simulink model "FDIlinkSimulinkSerial_20231225"  (R2022a)
settings: Solver=VariableStepAuto  StartTime=0.0  StopTime=inf  RelTol=1e-3
libraries: instrumentseriallib x2, aerolibconvert2 x1, sharedtransform x1
settings Model: Creator=JackyL  LastModifiedBy=Administrator
settings SolverCC: AlgebraicLoopSolver=TrustRegion
settings DataIOCC: ReturnWorkspaceOutputs=off
settings DebuggingCC: UnconnectedInputMsg=warning  UnconnectedOutputMsg=warning  UnconnectedLineMsg=warning  SFMachineParentedDataDiag=warning  ArithmeticOperatorsInVariantConditions=warning
settings SFSimCC: CustomCodeUndefinedFunction=UseInterfaceOnly
settings RTWCC: DLArmComputeVersion=19.05

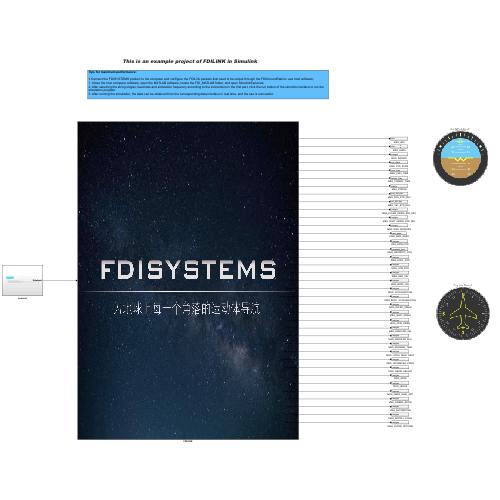
[thumbnail: Simulink's stored preview of the top-level diagram]
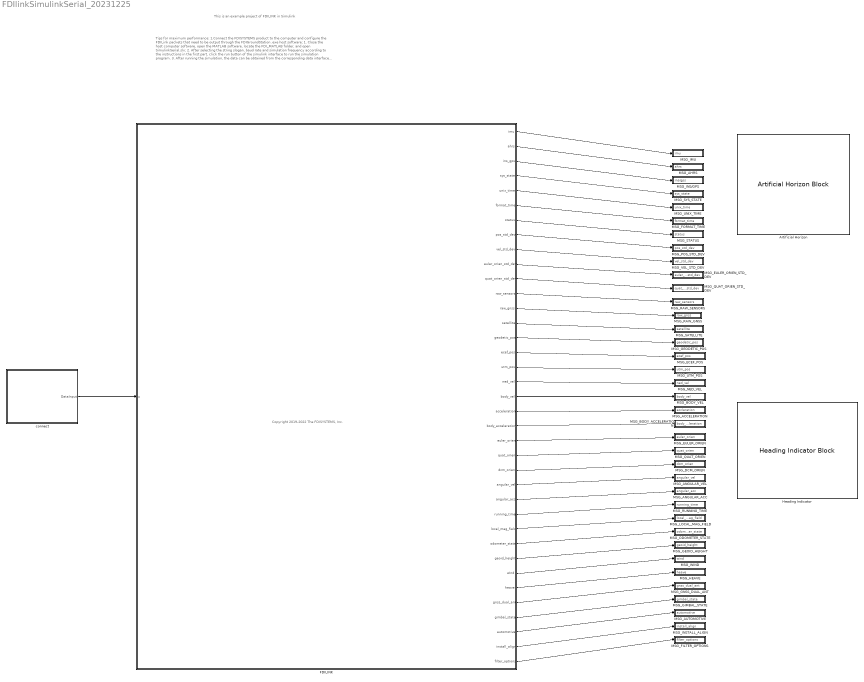
== system FDIlinkSimulinkSerial_20231225 ==
  note: This is an example project of FDILINK in Simulink
  note: Copyright 2019-2022 The FDISYSTEMS, Inc.
  note: Tips for maximum performance:
      |
      | 1.Connect the FDISYSTEMS product to the computer and configure the FDILink packets that need to be output through the FDIGroundStation .exe host software;
      | 1. Close the host computer software, open the MATLAB software, locate the FDI_MATLAB folder, and open SimulinkSerial.slx;
      | 2. After selecting the string slogan, baud rate and simulation frequency according to the instructions in the first part, click the run button of the simulink interface to run the simulation program.
      | 3. After running the simulation, the data can be obtained from the corresponding data interface in real time, and the use is successful.
      |
      | Secondary development: You can follow the example program in the following FDILINK module, add the data that needs to be parsed, specifically need to refer to the fdilink protocol document to write, and finally, pay attention to the computer software to enable this data frame.
  Artificial Horizon : ArtificialHorizonBlock
  FDILINK : MATLAB Function  TreatAsAtomicUnit=on
  Heading Indicator : HeadingIndicatorBlock
  MSG_ACCELERATION : Subsystem
  "MSG_AHRS " : Subsystem
  MSG_ANGULAR_ACC : Subsystem
  MSG_ANGULAR_VEL : Subsystem
  MSG_AUTOMOTIVE : Subsystem
  MSG_BODY_ACCELERATION : Subsystem
  MSG_BODY_VEL : Subsystem
  MSG_DCM_ORIEN : Subsystem
  MSG_ECEF_POS : Subsystem
  MSG_EULER_ORIEN : Subsystem
  MSG_EULER_ORIEN_STD_DEV : Subsystem
  MSG_FILTER_OPTIONS : Subsystem
  MSG_FORMAT_TIME : Subsystem
  MSG_GEODETIC_POS : Subsystem
  MSG_GEOID_HEIGHT : Subsystem
  MSG_GIMBAL_STATE : Subsystem
  MSG_GNSS_DUAL_ANT : Subsystem
  MSG_HEAVE : Subsystem
  "MSG_IMU " : Subsystem
  MSG_INS/GPS : Subsystem
  MSG_INSTALL_ALIGN : Subsystem
  MSG_LOCAL_MAG_FIELD : Subsystem
  MSG_NED_VEL : Subsystem
  MSG_ODOMETER_STATE : Subsystem
  MSG_POS_STD_DEV : Subsystem
  MSG_QUAT_ORIEN : Subsystem
  MSG_QUAT_ORIEN_STD_DEV : Subsystem
  MSG_RAW_GNSS : Subsystem
  MSG_RAW_SENSORS : Subsystem
  MSG_RUNNING_TIME : Subsystem
  MSG_SATELLITE : Subsystem
  MSG_STATUS : Subsystem
  MSG_SYS_STATE : Subsystem
  MSG_UNIX_TIME : Subsystem
  MSG_UTM_POS : Subsystem
  MSG_VEL_STD_DEV : Subsystem
  MSG_WIND : Subsystem
  connect : Subsystem
  wires:
  connect/1(DataInput) -> FDILINK/1(u)
  FDILINK/1(imu) -> "MSG_IMU "/1("imu ")
  FDILINK/2(ahrs) -> "MSG_AHRS "/1("ahrs ")
  FDILINK/3(ins_gps) -> MSG_INS/GPS/1("ins/gps ")
  FDILINK/13(raw_gnss) -> MSG_RAW_GNSS/1("raw_gnss ")
  FDILINK/15(geodetic_pos) -> MSG_GEODETIC_POS/1("geodetic_pos ")
  FDILINK/4(sys_state) -> MSG_SYS_STATE/1("sys_state ")
  FDILINK/5(unix_time) -> MSG_UNIX_TIME/1("unix_time ")
  FDILINK/6(format_time) -> MSG_FORMAT_TIME/1("format_time ")
  FDILINK/7(status) -> MSG_STATUS/1("status ")
  FDILINK/8(pos_std_dev) -> MSG_POS_STD_DEV/1("pos_std_dev ")
  FDILINK/9(vel_std_dev) -> MSG_VEL_STD_DEV/1("vel_std_dev ")
  FDILINK/10(euler_orien_std_dev) -> MSG_EULER_ORIEN_STD_DEV/1("euler_orien_std_dev ")
  FDILINK/11(quat_orien_std_dev) -> MSG_QUAT_ORIEN_STD_DEV/1("quat_orien_std_dev ")
  FDILINK/12(raw_sensors) -> MSG_RAW_SENSORS/1("raw_sensors ")
  FDILINK/14(satellite) -> MSG_SATELLITE/1("satellite ")
  FDILINK/16(ecef_pos) -> MSG_ECEF_POS/1("ecef_pos ")
  FDILINK/17(utm_pos) -> MSG_UTM_POS/1("utm_pos ")
  FDILINK/18(ned_vel) -> MSG_NED_VEL/1("ned_vel ")
  FDILINK/19(body_vel) -> MSG_BODY_VEL/1("body_vel ")
  FDILINK/20(acceleration) -> MSG_ACCELERATION/1("accleration ")
  FDILINK/21(body_acceleration) -> MSG_BODY_ACCELERATION/1("body_acceleration ")
  FDILINK/22(euler_orien) -> MSG_EULER_ORIEN/1("euler_orien ")
  FDILINK/23(quat_orien) -> MSG_QUAT_ORIEN/1("quat_orien ")
  FDILINK/24(dcm_orien) -> MSG_DCM_ORIEN/1("dcm_orien ")
  FDILINK/25(angular_vel) -> MSG_ANGULAR_VEL/1("angular_vel ")
  FDILINK/26(angular_acc) -> MSG_ANGULAR_ACC/1("angular_acc ")
  FDILINK/27(running_time) -> MSG_RUNNING_TIME/1("running_time ")
  FDILINK/28(local_mag_field) -> MSG_LOCAL_MAG_FIELD/1("local_mag_field ")
  FDILINK/29(odometer_state) -> MSG_ODOMETER_STATE/1("odometer_state ")
  FDILINK/30(geoid_height) -> MSG_GEOID_HEIGHT/1("geoid_height ")
  FDILINK/31(wind) -> MSG_WIND/1("wind ")
  FDILINK/32(heave) -> MSG_HEAVE/1("heave ")
  FDILINK/33(gnss_dual_ant) -> MSG_GNSS_DUAL_ANT/1("gnss_dual_ant ")
  FDILINK/34(gimbal_state) -> MSG_GIMBAL_STATE/1("gimbal_state ")
  FDILINK/35(automotive) -> MSG_AUTOMOTIVE/1("automotive ")
  FDILINK/36(install_align) -> MSG_INSTALL_ALIGN/1("install_align ")
  FDILINK/37(filter_options) -> MSG_FILTER_OPTIONS/1("filter_options ")

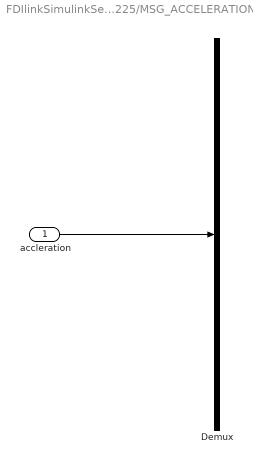
== system FDIlinkSimulinkSerial_20231225/MSG_ACCELERATION ==
  "accleration " : Inport
  Demux : Demux  Outputs=3
  wires:
  "accleration "/1 -> Demux/1

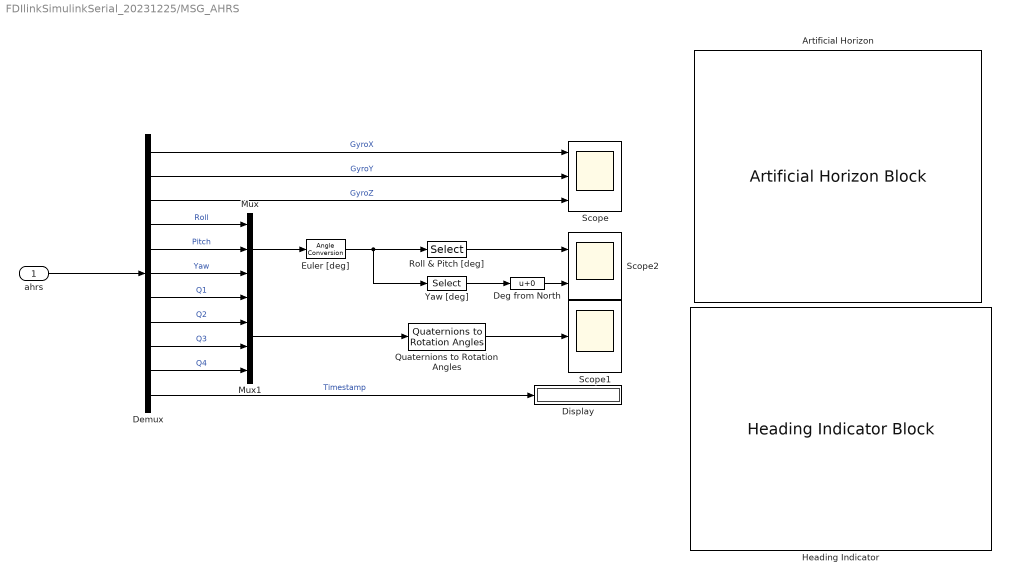
== system FDIlinkSimulinkSerial_20231225/MSG_AHRS  ==
  "ahrs " : Inport
  Artificial Horizon : ArtificialHorizonBlock
  Deg from North : Bias  SaturateOnIntegerOverflow=off
  Demux : Demux  Outputs=11
  Display : Display
  Euler [deg] : aerolibconvert2/Angle Conversion  IU=rad  OU=deg
  Heading Indicator : HeadingIndicatorBlock
  Mux : Mux  Inputs=3
  Mux1 : Mux
  Quaternions to Rotation Angles : sharedtransform/Quaternions to Rotation Angles  rotationOrder=ZYX  aMode=aMode
      settings: SourceProductBaseCode=AE,PW,DR,MT,VE
  Roll & Pitch [deg] : Selector  InputPortWidth=3  IndexOptions=Index vector (dialog)  Indices=[1 2]  OutputSizes=1
  Scope : Scope  NumInputPorts=3
  Scope1 : Scope
  Scope2 : Scope  NumInputPorts=2
  Yaw [deg] : Selector  InputPortWidth=3  IndexOptions=Index vector (dialog)  Indices=[3]  OutputSizes=1
  wires:
  "ahrs "/1 -> Demux/1
  Demux/1 -> Scope/1  "GyroX"
  Demux/2 -> Scope/2  "GyroY"
  Demux/3 -> Scope/3  "GyroZ"
  Demux/5 -> Mux/2  "Pitch"
  Demux/7 -> Mux1/1  "Q1"
  Demux/8 -> Mux1/2  "Q2"
  Demux/9 -> Mux1/3  "Q3"
  Demux/10 -> Mux1/4  "Q4"
  Demux/11 -> Display/1  "Timestamp"
  Demux/4 -> Mux/1  "Roll"
  Demux/6 -> Mux/3  "Yaw"
  Mux/1 -> Euler [deg]/1
  Euler [deg]/1 -> Yaw [deg]/1, Roll & Pitch [deg]/1
  Yaw [deg]/1 -> Deg from North/1
  Mux1/1 -> Quaternions to Rotation Angles/1
  Quaternions to Rotation Angles/1 -> Scope1/1
  Roll & Pitch [deg]/1 -> Scope2/1
  Deg from North/1 -> Scope2/2

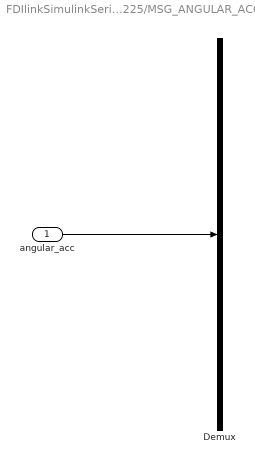
== system FDIlinkSimulinkSerial_20231225/MSG_ANGULAR_ACC ==
  "angular_acc " : Inport
  Demux : Demux  Outputs=3
  wires:
  "angular_acc "/1 -> Demux/1

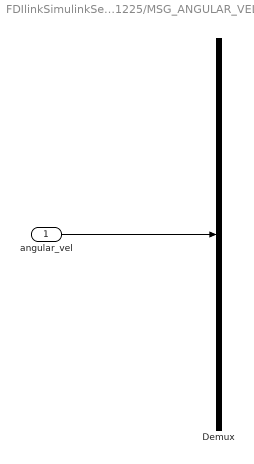
== system FDIlinkSimulinkSerial_20231225/MSG_ANGULAR_VEL ==
  "angular_vel " : Inport
  Demux : Demux  Outputs=3
  wires:
  "angular_vel "/1 -> Demux/1

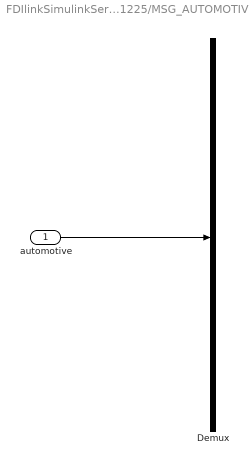
== system FDIlinkSimulinkSerial_20231225/MSG_AUTOMOTIVE ==
  "automotive " : Inport
  Demux : Demux  Outputs=6
  wires:
  "automotive "/1 -> Demux/1

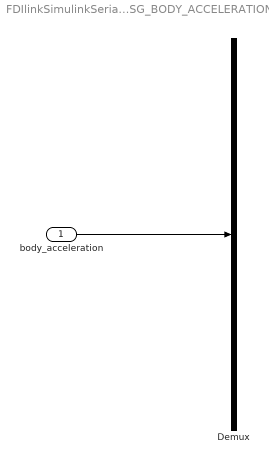
== system FDIlinkSimulinkSerial_20231225/MSG_BODY_ACCELERATION ==
  "body_acceleration " : Inport
  Demux : Demux
  wires:
  "body_acceleration "/1 -> Demux/1

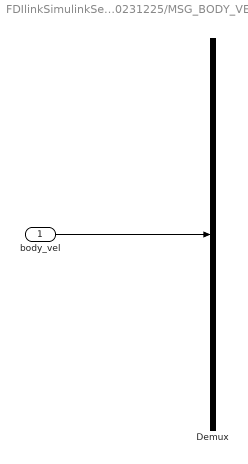
== system FDIlinkSimulinkSerial_20231225/MSG_BODY_VEL ==
  "body_vel " : Inport
  Demux : Demux  Outputs=3
  wires:
  "body_vel "/1 -> Demux/1

== system FDIlinkSimulinkSerial_20231225/MSG_DCM_ORIEN ==
  "dcm_orien " : Inport
  Demux : Demux  Outputs=9
  wires:
  "dcm_orien "/1 -> Demux/1

== system FDIlinkSimulinkSerial_20231225/MSG_ECEF_POS ==
  "ecef_pos " : Inport
  Demux : Demux  Outputs=3
  wires:
  "ecef_pos "/1 -> Demux/1

== system FDIlinkSimulinkSerial_20231225/MSG_EULER_ORIEN ==
  "euler_orien " : Inport
  Demux : Demux  Outputs=3
  wires:
  "euler_orien "/1 -> Demux/1

== system FDIlinkSimulinkSerial_20231225/MSG_EULER_ORIEN_STD_DEV ==
  "euler_orien_std_dev " : Inport
  Demux : Demux  Outputs=3
  wires:
  "euler_orien_std_dev "/1 -> Demux/1

== system FDIlinkSimulinkSerial_20231225/MSG_FILTER_OPTIONS ==
  "filter_options " : Inport
  Demux : Demux  Outputs=21
  wires:
  "filter_options "/1 -> Demux/1

== system FDIlinkSimulinkSerial_20231225/MSG_FORMAT_TIME ==
  "format_time " : Inport
  Demux : Demux  Outputs=9
  wires:
  "format_time "/1 -> Demux/1

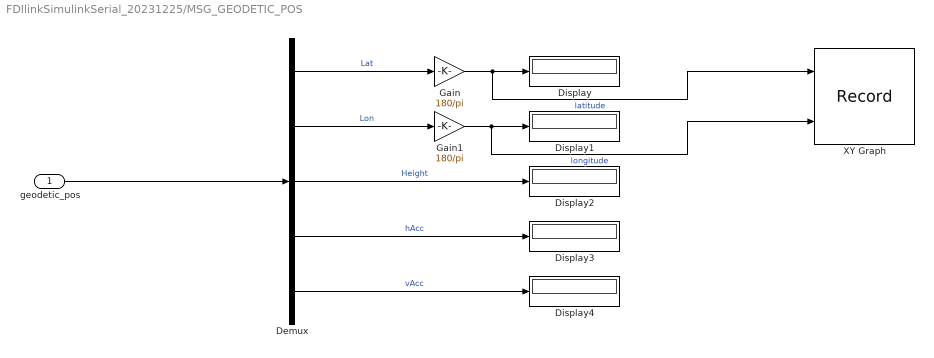
== system FDIlinkSimulinkSerial_20231225/MSG_GEODETIC_POS ==
  "geodetic_pos " : Inport
  Demux : Demux  Outputs=5
  Display{,1..4} (5 alike) : Display
  Gain : Gain  Gain=180/pi
  Gain1 : Gain  Gain=180/pi
  XY Graph : Record  FileSettingsInternal="{\"entries\":[{\"content\":{\"excelSettings\":{\"content\":{},\"type\":\"Streamout.ExcelSettings\"}},\"type\":\"Streamout.FileSettingStorage\",\"uuid\":\"c57b3c35-ac54-404b-860e-26f47809a26e\"}],\"packageUris\":[\"http://schema.mathworks.com/mf0/streamout_blocks/R2020a\"],\"version\":\"1.0\"}"  Layout=[1 1]  SignalsInternal="{\"entries\":[{\"content\":{\"signals\":[{\"content\":{\"blockPath\":[\"FDIlinkSimulinkSerial_2023/MSG_GEODETIC_POS/XY Graph\"],\"channel\":[],\"dimensions\":[1],\"domain\":\"FDIlinkSimulinkSerial_2023/MSG_GEODETIC_POS/XY Graph\",\"lineColor\":\"#a2142f\",\"plots\":[1],\"port\":1,\"sid\":[\"\"],\"signalID\":52640,\"signalName\":\"latitude\"},\"type\":\"RecordBlkView.Signal\",\"uuid\":\"bd247451-c40f-4c59-b5e0-45e0f2542574\"},{\"content\":{\"blockPath\":[\"FDIlinkSimulinkSerial_2023/MSG_GEODETIC_POS/XY Graph\"],\"channel\":[],\"dimensions\":[1],\"domain\":\"FDIlinkSimulinkSerial_2023/MSG_GEODETIC_POS/XY Graph\",\"lineColor\":\"#139fff\",\"plots\":[1],\"port\":2,\"sid\":[\"\"],\"signalID\":52644,\"signalName\":\"longitude\"},\"type\":\"RecordBlkView.Signal\",\"uuid\":\"75755b6a-9d0c-4554-936c-c924832028f1\"}]},\"type\":\"RecordBlkView.InputSignals\",\"uuid\":\"5899f446-d7af-45c7-ad3b-5777b81863a8\"}],\"packageUris\":[\"http://schema.mathworks.com/mf0/streamout_blocks/R2020a\"],\"version\":\"1.0\"}"  VisualizationBindings="{\"mapsplugin\":{\"info\":[{\"bindingParametersList\":[{\"parameter\":\"Latitude\",\"signalID\":52640,\"signalName\":\"latitude\"},{\"parameter\":\"Longitude\",\"signalID\":52644,\"signalName\":\"longitude\"}],\"subplotID\":1}]}}"  CompatibilityTag=XY
  wires:
  "geodetic_pos "/1 -> Demux/1
  Demux/1 -> Gain/1  "Lat"
  Demux/3 -> Display2/1  "Height"
  Demux/4 -> Display3/1  "hAcc"
  Demux/2 -> Gain1/1  "Lon"
  Gain/1 -> XY Graph/1, Display/1  "latitude"
  Gain1/1 -> XY Graph/2, Display1/1  "longitude"
  Demux/5 -> Display4/1  "vAcc"

== system FDIlinkSimulinkSerial_20231225/MSG_GEOID_HEIGHT ==
  "geoid_height " : Inport
  Demux : Demux  Outputs=1
  wires:
  "geoid_height "/1 -> Demux/1

== system FDIlinkSimulinkSerial_20231225/MSG_GIMBAL_STATE ==
  "gimbal_state " : Inport
  Demux : Demux  Outputs=2
  wires:
  "gimbal_state "/1 -> Demux/1

== system FDIlinkSimulinkSerial_20231225/MSG_GNSS_DUAL_ANT ==
  "gnss_dual_ant " : Inport
  Demux : Demux  Outputs=23
  wires:
  "gnss_dual_ant "/1 -> Demux/1

== system FDIlinkSimulinkSerial_20231225/MSG_HEAVE ==
  "heave " : Inport
  Demux : Demux
  wires:
  "heave "/1 -> Demux/1

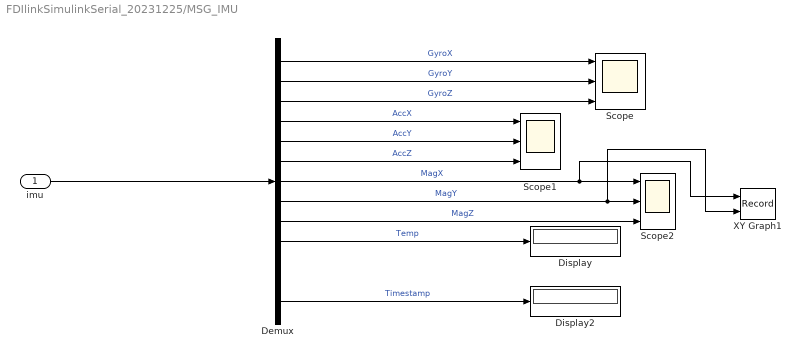
== system FDIlinkSimulinkSerial_20231225/MSG_IMU  ==
  "imu " : Inport
  Demux : Demux  Outputs=13
  Display : Display
  Display2 : Display
  Scope : Scope  NumInputPorts=3
  Scope1 : Scope  NumInputPorts=3
  Scope2 : Scope  NumInputPorts=3
  XY Graph1 : Record  FileSettingsInternal="{\"entries\":[{\"content\":{\"excelSettings\":{\"content\":{},\"type\":\"Streamout.ExcelSettings\"}},\"type\":\"Streamout.FileSettingStorage\",\"uuid\":\"65ec4354-fc0c-4555-b10d-ce23bbae165b\"}],\"packageUris\":[\"http://schema.mathworks.com/mf0/streamout_blocks/R2020a\"],\"version\":\"1.0\"}"  Layout=[1 1]  SignalsInternal="{\"entries\":[{\"content\":{\"signals\":[{\"content\":{\"blockPath\":[\"FDIlinkSimulinkSerial_2023/MSG_IMU /XY Graph1\"],\"channel\":[],\"dimensions\":[1],\"domain\":\"FDIlinkSimulinkSerial_2023/MSG_IMU /XY Graph1\",\"lineColor\":\"#edb120\",\"plots\":[1],\"port\":1,\"sid\":[\"\"],\"signalID\":52648,\"signalName\":\"MagX\"},\"type\":\"RecordBlkView.Signal\",\"uuid\":\"e399e0cc-c2a5-4ba5-86a0-381cf1e076fb\"},{\"content\":{\"blockPath\":[\"FDIlinkSimulinkSerial_2023/MSG_IMU /XY Graph1\"],\"channel\":[],\"dimensions\":[1],\"domain\":\"FDIlinkSimulinkSerial_2023/MSG_IMU /XY Graph1\",\"lineColor\":\"#7e2f8e\",\"plots\":[1],\"port\":2,\"sid\":[\"\"],\"signalID\":52652,\"signalName\":\"MagY\"},\"type\":\"RecordBlkView.Signal\",\"uuid\":\"577b7574-98dc-4594-a01f-2f18dd9d9adf\"}]},\"type\":\"RecordBlkView.InputSignals\",\"uuid\":\"5e8bd6d5-46a9-48a2-996e-792b251aa4c2\"}],\"packageUris\":[\"http://schema.mathworks.com/mf0/streamout_blocks/R2020a\"],\"version\":\"1.0\"}"  VisualizationBindings="{\"xyplotplugin\":{\"info\":[{\"series\":[{\"bindingParametersList\":[{\"parameter\":\"Y-Axis\",\"signalID\":52652,\"signalName\":\"MagY\"},{\"parameter\":\"X-Axis\",\"signalID\":52648,\"signalName\":\"MagX\"}],\"seriesID\":49908}],\"subplotID\":1}]}}"  CompatibilityTag=XY
  wires:
  "imu "/1 -> Demux/1
  Demux/2 -> Scope/2  "GyroY"
  Demux/10 -> Display/1  "Temp"
  Demux/8 -> XY Graph1/2, Scope2/2  "MagY"
  Demux/5 -> Scope1/2  "AccY"
  Demux/7 -> XY Graph1/1, Scope2/1  "MagX"
  Demux/6 -> Scope1/3  "AccZ"
  Demux/9 -> Scope2/3  "MagZ"
  Demux/3 -> Scope/3  "GyroZ"
  Demux/4 -> Scope1/1  "AccX"
  Demux/1 -> Scope/1  "GyroX"
  Demux/13 -> Display2/1  "Timestamp"

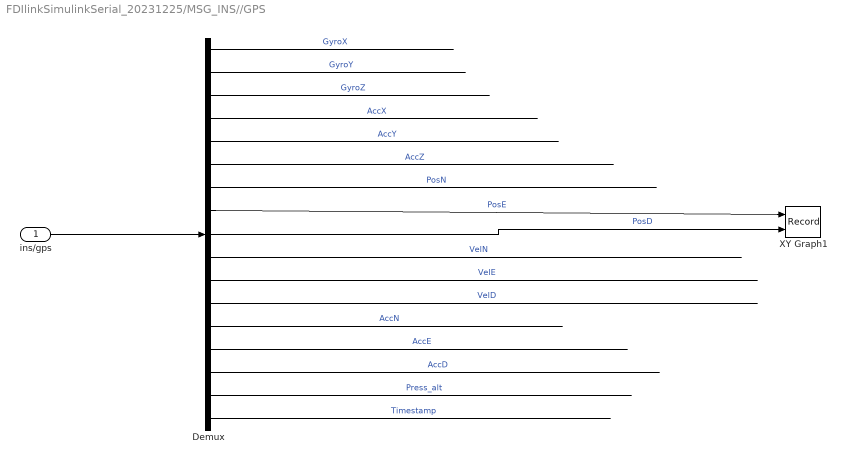
== system FDIlinkSimulinkSerial_20231225/MSG_INS//GPS ==
  "ins/gps " : Inport
  Demux : Demux  Outputs=17
  XY Graph1 : Record  FileSettingsInternal="{\"entries\":[{\"content\":{\"excelSettings\":{\"content\":{},\"type\":\"Streamout.ExcelSettings\"}},\"type\":\"Streamout.FileSettingStorage\",\"uuid\":\"c1e5a542-af21-46d7-be2d-958286783f12\"}],\"packageUris\":[\"http://schema.mathworks.com/mf0/streamout_blocks/R2020a\"],\"version\":\"1.0\"}"  Layout=[1 1]  SignalsInternal="{\"entries\":[{\"content\":{\"signals\":[{\"content\":{\"blockPath\":[\"FDIlinkSimulinkSerial_2023/MSG_INS//GPS/XY Graph1\"],\"channel\":[],\"dimensions\":[1],\"domain\":\"FDIlinkSimulinkSerial_2023/MSG_INS//GPS/XY Graph1\",\"lineColor\":\"#ff13a6\",\"plots\":[1],\"port\":1,\"sid\":[\"\"],\"signalID\":52656,\"signalName\":\"PosE\"},\"type\":\"RecordBlkView.Signal\",\"uuid\":\"021f53f5-616b-4887-be3d-6d5316776099\"},{\"content\":{\"blockPath\":[\"FDIlinkSimulinkSerial_2023/MSG_INS//GPS/XY Graph1\"],\"channel\":[],\"dimensions\":[1],\"domain\":\"FDIlinkSimulinkSerial_2023/MSG_INS//GPS/XY Graph1\",\"lineColor\":\"#fe330a\",\"plots\":[1],\"port\":2,\"sid\":[\"\"],\"signalID\":52660,\"signalName\":\"PosD\"},\"type\":\"RecordBlkView.Signal\",\"uuid\":\"6068f2ee-5e6c-42f1-978f-d58a864ce9d3\"}]},\"type\":\"RecordBlkView.InputSignals\",\"uuid\":\"c5067fb9-dce5-4b7d-8ad8-81806b3f26c2\"}],\"packageUris\":[\"http://schema.mathworks.com/mf0/streamout_blocks/R2020a\"],\"version\":\"1.0\"}"  VisualizationBindings="{\"xyplotplugin\":{\"info\":[{\"series\":[{\"bindingParametersList\":[{\"parameter\":\"X-Axis\",\"signalID\":52656,\"signalName\":\"PosE\"},{\"parameter\":\"Y-Axis\",\"signalID\":52660,\"signalName\":\"PosD\"}],\"seriesID\":13281}],\"subplotID\":1}]}}"  CompatibilityTag=XY
  wires:
  "ins/gps "/1 -> Demux/1
  Demux/1 -> ?  "GyroX"
  Demux/2 -> ?  "GyroY"
  Demux/3 -> ?  "GyroZ"
  Demux/4 -> ?  "AccX"
  Demux/5 -> ?  "AccY"
  Demux/6 -> ?  "AccZ"
  Demux/7 -> ?  "PosN"
  Demux/8 -> XY Graph1/1  "PosE"
  Demux/9 -> XY Graph1/2  "PosD"
  Demux/10 -> ?  "VelN"
  Demux/11 -> ?  "VelE"
  Demux/12 -> ?  "VelD"
  Demux/13 -> ?  "AccN"
  Demux/14 -> ?  "AccE"
  Demux/15 -> ?  "AccD"
  Demux/16 -> ?  "Press_alt"
  Demux/17 -> ?  "Timestamp"

== system FDIlinkSimulinkSerial_20231225/MSG_INSTALL_ALIGN ==
  "install_align " : Inport
  Demux : Demux  Outputs=11
  wires:
  "install_align "/1 -> Demux/1

== system FDIlinkSimulinkSerial_20231225/MSG_LOCAL_MAG_FIELD ==
  "local_mag_field " : Inport
  Demux : Demux  Outputs=6
  wires:
  "local_mag_field "/1 -> Demux/1

== system FDIlinkSimulinkSerial_20231225/MSG_NED_VEL ==
  "ned_vel " : Inport
  Demux : Demux  Outputs=3
  wires:
  "ned_vel "/1 -> Demux/1

== system FDIlinkSimulinkSerial_20231225/MSG_ODOMETER_STATE ==
  "odometer_state " : Inport
  Demux : Demux  Outputs=6
  wires:
  "odometer_state "/1 -> Demux/1

== system FDIlinkSimulinkSerial_20231225/MSG_POS_STD_DEV ==
  "pos_std_dev " : Inport
  Demux : Demux  Outputs=3
  wires:
  "pos_std_dev "/1 -> Demux/1

== system FDIlinkSimulinkSerial_20231225/MSG_QUAT_ORIEN ==
  "quat_orien " : Inport
  Demux : Demux
  wires:
  "quat_orien "/1 -> Demux/1

== system FDIlinkSimulinkSerial_20231225/MSG_QUAT_ORIEN_STD_DEV ==
  "quat_orien_std_dev " : Inport
  Demux : Demux
  wires:
  "quat_orien_std_dev "/1 -> Demux/1

== system FDIlinkSimulinkSerial_20231225/MSG_RAW_GNSS ==
  "raw_gnss " : Inport
  Demux : Demux  Outputs=13
  wires:
  "raw_gnss "/1 -> Demux/1

== system FDIlinkSimulinkSerial_20231225/MSG_RAW_SENSORS ==
  "raw_sensors " : Inport
  Demux : Demux  Outputs=12
  wires:
  "raw_sensors "/1 -> Demux/1

== system FDIlinkSimulinkSerial_20231225/MSG_RUNNING_TIME ==
  "running_time " : Inport
  Demux : Demux  Outputs=2
  wires:
  "running_time "/1 -> Demux/1

== system FDIlinkSimulinkSerial_20231225/MSG_SATELLITE ==
  "satellite " : Inport
  Demux : Demux  Outputs=3
  wires:
  "satellite "/1 -> Demux/1

== system FDIlinkSimulinkSerial_20231225/MSG_STATUS ==
  "status " : Inport
  Demux : Demux  Outputs=2
  wires:
  "status "/1 -> Demux/1

== system FDIlinkSimulinkSerial_20231225/MSG_SYS_STATE ==
  "sys_state " : Inport
  Demux : Demux  Outputs=23
  wires:
  "sys_state "/1 -> Demux/1

== system FDIlinkSimulinkSerial_20231225/MSG_UNIX_TIME ==
  "unix_time " : Inport
  Demux : Demux  Outputs=2
  wires:
  "unix_time "/1 -> Demux/1

== system FDIlinkSimulinkSerial_20231225/MSG_UTM_POS ==
  "utm_pos " : Inport
  Demux : Demux  Outputs=5
  wires:
  "utm_pos "/1 -> Demux/1

== system FDIlinkSimulinkSerial_20231225/MSG_VEL_STD_DEV ==
  "vel_std_dev " : Inport
  Demux : Demux  Outputs=3
  wires:
  "vel_std_dev "/1 -> Demux/1

== system FDIlinkSimulinkSerial_20231225/MSG_WIND ==
  "wind " : Inport
  Demux : Demux  Outputs=3
  wires:
  "wind "/1 -> Demux/1

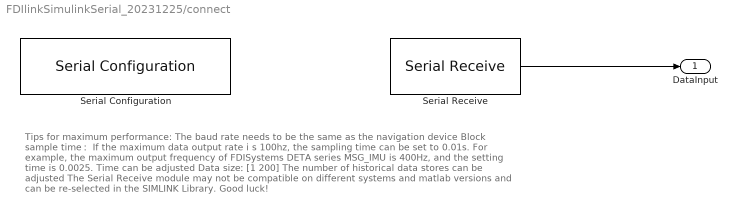
== system FDIlinkSimulinkSerial_20231225/connect ==
  note: Tips for maximum performance:
      |
      | The baud rate needs to be the same as the navigation device
      | Block sample time： If the maximum data output rate i s 100hz, the sampling time can be set to 0.01s. For example, the maximum output frequency of FDISystems DETA series MSG_IMU is 400Hz, and the setting time is 0.0025. Time can be adjusted
      | Data size：[1 200] The number of historical data stores can be adjusted
      | The Serial Receive module may not be compatible on different systems and matlab versions and can be re-selected in the SIMLINK Library. Good luck!
  Serial Configuration : instrumentseriallib/Serial Configuration  Priority=-200000  PortSel=COM22  Port=COM22  ComPort=COM22  BaudRate=921600  DataBits=8  Parity=none  StopBits=1  ByteOrder=little-endian  FlowControl=none  Timeout=10  SimulateUsing=Interpreted execution  BlockInModel=on  aMode=1
      settings: SourceProductBaseCode=OT,IC,MT
  Serial Receive : instrumentseriallib/Serial Receive  Priority=1  PortSel=COM22  Port=COM22  ComPort=COM22  DataType=uint8  SaveDataType=uint8  ToggleHeader=off  Header=[]  ToggleTerminator=off  Terminator=<none>  CustomTerminator=[]  InputFormat=Column major  ToggleDataSize=on  DataSize=[1 200]  EnableBlockingMode=on  ActionDataUnavailable=Output last received value  ActionWhenDataUnavailable=Output last received value  CustomValue=0  SampleTime=0.01  SimulateUsing=Interpreted execution  BlockInModel=on  aMode=1
      settings: SourceProductBaseCode=OT,IC,MT
  DataInput : Outport
  wires:
  Serial Receive/1 -> DataInput/1

== matlab function FDIlinkSimulinkSerial_20231225/FDILINK ==
  data: imu output; u input; ahrs output; ins_gps output; sys_state output; unix_time output; format_time output; status output; pos_std_dev output; vel_std_dev output; euler_orien_std_dev output; quat_orien_std_dev output; raw_sensors output; raw_gnss output; satellite output; geodetic_pos output; ecef_pos output; utm_pos output; ned_vel output; body_vel output; acceleration output; body_acceleration output; euler_orien output; quat_orien output; dcm_orien output; angular_vel output; angular_acc output; running_time output; local_mag_field output; odometer_state output; geoid_height output; wind output; heave output; gnss_dual_ant output; gimbal_state output; automotive output; install_align output; filter_options output
%% Describes decoding FDILink communication protocol data frames in MATLAB & simulink
% You can follow the example program in the following FDILINK module,
% add the data that needs to be parsed, specifically need to refer to the fdilink protocol document to write,
% and finally, pay attention to the computer software to enable this data frame.

% Copyright 2019-2021 The FDISYSTEMS, Inc.

function [imu,ahrs,ins_gps,sys_state,unix_time,format_time,status,pos_std_dev,vel_std_dev,euler_orien_std_dev,quat_orien_std_dev,raw_sensors,raw_gnss,satellite,geodetic_pos,ecef_pos,utm_pos,ned_vel,body_vel,acceleration,...
    body_acceleration,euler_orien,quat_orien,dcm_orien,angular_vel,angular_acc,running_time,local_mag_field,odometer_state,geoid_height,wind,heave,gnss_dual_ant,gimbal_state,automotive,install_align,filter_options] = fcn(u)
persistent FStatus;
persistent ReceiveDataLeft;
persistent ReceiveType;
persistent Buffer;
persistent BufferIndex;
persistent lastimu;
persistent lastahrs;
persistent lastins_Gps;
persistent lastsys_state;
persistent lastunix_time;
persistent lastformat_time;
persistent laststatus;
persistent lastpos_std_dev;
persistent lastvel_std_dev;
persistent lasteuler_orien_std_dev;
persistent lastquat_orien_std_dev;
persistent lastraw_sensors;
persistent lastraw_gnss;
persistent lastsatellite;
persistent lastgeodetic_pos;
persistent lastecef_pos;
persistent lastutm_pos;
persistent lastned_vel;
persistent lastbody_vel;
persistent lastacceleration;
persistent lastbody_acceleration;
persistent lasteuler_orien;
persistent lastquat_orien;
persistent lastdcm_orien;
persistent lastangular_vel;
persistent lastangular_acc;
persistent lastrunning_time;
persistent lastlocal_mag_field;
persistent lastodometer_state;
persistent lastgeoid_height;
persistent lastwind;
persistent lastheave;
persistent lastgnss_dual_ant;
persistent lastgimbal_state;
persistent lastautomotive;
persistent lastinstall_align;
persistent lastfilter_options;

if isempty(FStatus)
    FStatus = 0;
    ReceiveDataLeft = uint8(0);
    BufferIndex = uint8(0);
    Buffer = uint8(zeros(1,256));
    ReceiveType = uint8(0);
    lastimu  = zeros(13,1);
    lastahrs = zeros(11,1);
    lastins_Gps = zeros(17,1);
    lastsys_state  = zeros(23,1);
    lastunix_time = zeros(2,1);
    lastformat_time = zeros(9,1);
    laststatus  = zeros(2,1);
    lastpos_std_dev = zeros(3,1);
    lastvel_std_dev = zeros(3,1);
    lasteuler_orien_std_dev  = zeros(3,1);
    lastquat_orien_std_dev = zeros(4,1);
    lastraw_sensors = zeros(12,1);
    lastraw_gnss  = zeros(13,1);
    lastsatellite = zeros(3,1);
    lastgeodetic_pos = zeros(5,1);
    lastecef_pos  = zeros(3,1);
    lastutm_pos = zeros(5,1);
    lastned_vel = zeros(3,1);
    lastbody_vel  = zeros(3,1);
    lastacceleration = zeros(3,1);
    lastbody_acceleration = zeros(4,1);
    lasteuler_orien  = zeros(3,1);
    lastquat_orien = zeros(4,1);
    lastdcm_orien = zeros(9,1);
    lastangular_vel  = zeros(3,1);
    lastangular_acc = zeros(3,1);
    lastrunning_time = zeros(2,1);
    lastlocal_mag_field  = zeros(6,1);
    lastodometer_state = zeros(6,1);
    lastgeoid_height = zeros(1,1);
    lastwind  = zeros(3,1);
    lastheave = zeros(4,1);
    lastgnss_dual_ant = zeros(23,1);
    lastgimbal_state  = zeros(2,1);
    lastautomotive = zeros(6,1);
    lastinstall_align = zeros(11,1);
    lastfilter_options = zeros(21,1);

end
%数据帧帧头FC
SerialBoot_STX_Flag = uint8(252);
%数据帧帧尾FD
SerialBoot_EDX_Flag = uint8(253);
for i = 1:length(u)
    value = u(i);
    switch (FStatus)
        case 0
            ReceiveDataLeft = uint8(0);
            if value == SerialBoot_STX_Flag
                FStatus = 1;
            end
        case 1
            %ReceiveType对应数据帧里的指令类别，比如IMU数据包为0x40，AHRS数据包为0x41，转化为十进制就是64和65；
            ReceiveType = value;
            FStatus = 2;
        case 2
            %ReceiveDataLeft对应数据帧里的暂未复制带Buffer里的数据长度（位），此时被赋予的值对应该数据包完整的数据长度；
            ReceiveDataLeft = value;
            BufferIndex = uint8(1);
            FStatus = 3;
        case 3
            FStatus = 4;
        case 4
            if ReceiveDataLeft == 0
                FStatus = 0;
            else
                FStatus = 5;
            end
        case 5
            FStatus = 6;
        case 6
            FStatus = 7;
        case 7
            %对应数据帧里的载荷，此时Buffer数据按顺序存储载荷里的数据直到全部复制完成
            Buffer(BufferIndex) = value;
            BufferIndex = BufferIndex + 1;
            ReceiveDataLeft = ReceiveDataLeft - 1;
            if ReceiveDataLeft == 0
                FStatus = 8;
            end
        case 8
            if (value == SerialBoot_EDX_Flag)
                switch(ReceiveType)
                    case 64
                        %% 解析MSG_IMU
                        lastimu(1) = typecast(Buffer(1:4),'single');
                        lastimu(2) = typecast(Buffer(5:8),'single');
                        lastimu(3) = typecast(Buffer(9:12),'single');
                        lastimu(4) = typecast(Buffer(13:16),'single');
                        lastimu(5) = typecast(Buffer(17:20),'single');
                        lastimu(6) = typecast(Buffer(21:24),'single');
                        lastimu(7) = typecast(Buffer(25:28),'single');
                        lastimu(8) = typecast(Buffer(29:32),'single');
                        lastimu(9) = typecast(Buffer(33:36),'single');
                        lastimu(10) = typecast(Buffer(37:40),'single');
                        lastimu(11) = typecast(Buffer(41:44),'single');
                        lastimu(12) = typecast(Buffer(45:48),'single');
                        lastimu(13) = typecast(Buffer(49:56),'uint64');
                    case 65
                        %% 解析MSG_AHRS
                        lastahrs(1) = typecast(Buffer(1:4),'single');
                        lastahrs(2) = typecast(Buffer(5:8),'single');
                        lastahrs(3) = typecast(Buffer(9:12),'single');
                        lastahrs(4) = typecast(Buffer(13:16),'single');
                        lastahrs(5) = typecast(Buffer(17:20),'single');
                        lastahrs(6) = typecast(Buffer(21:24),'single');
                        lastahrs(7) = typecast(Buffer(25:28),'single');
                        lastahrs(8) = typecast(Buffer(29:32),'single');
                        lastahrs(9) = typecast(Buffer(33:36),'single');
                        lastahrs(10) = typecast(Buffer(37:40),'single');
                        lastahrs(11) = typecast(Buffer(41:48),'uint64');
                    case 66
                        %% 解析MSG_INS/GPS
                        lastins_Gps(1) = typecast(Buffer(1:4),'single');
                        lastins_Gps(2) = typecast(Buffer(5:8),'single');
                        lastins_Gps(3) = typecast(Buffer(9:12),'single');
                        lastins_Gps(4) = typecast(Buffer(13:16),'single');
                        lastins_Gps(5) = typecast(Buffer(17:20),'single');
                        lastins_Gps(6) = typecast(Buffer(21:24),'single');
                        lastins_Gps(7) = typecast(Buffer(25:28),'single');
                        lastins_Gps(8) = typecast(Buffer(29:32),'single');
                        lastins_Gps(9) = typecast(Buffer(33:36),'single');
                        lastins_Gps(10) = typecast(Buffer(37:40),'single');
                        lastins_Gps(11) = typecast(Buffer(41:44),'single');
                        lastins_Gps(12) = typecast(Buffer(45:48),'single');
                        lastins_Gps(13) = typecast(Buffer(49:52),'single');
                        lastins_Gps(14) = typecast(Buffer(53:56),'single');
                        lastins_Gps(15) = typecast(Buffer(57:60),'single');
                        lastins_Gps(16) = typecast(Buffer(61:64),'single');
                        lastins_Gps(17) = typecast(Buffer(65:72),'uint64');
                    case 80
                        %% 解析MSG_SYS_STATE
                        lastsys_state(1) = typecast(Buffer(1:2),'uint16');
                        lastsys_state(2) = typecast(Buffer(3:4),'uint16');
                        lastsys_state(3) = typecast(Buffer(5:8),'uint32');
                        lastsys_state(4) = typecast(Buffer(9:12),'uint32');
                        lastsys_state(5) = typecast(Buffer(13:20),'double');
                        lastsys_state(6) = typecast(Buffer(21:28),'double');
                        lastsys_state(7) = typecast(Buffer(29:36),'double');
                        lastsys_state(8) = typecast(Buffer(37:40),'single');
                        lastsys_state(9) = typecast(Buffer(41:44),'single');
                        lastsys_state(10) = typecast(Buffer(45:48),'single');
                        lastsys_state(11) = typecast(Buffer(49:52),'single');
                        lastsys_state(12) = typecast(Buffer(53:56),'single');
                        lastsys_state(13) = typecast(Buffer(57:60),'single');
                        lastsys_state(14) = typecast(Buffer(61:64),'single');
                        lastsys_state(15) = typecast(Buffer(65:68),'single');
                        lastsys_state(16) = typecast(Buffer(69:72),'single');
                        lastsys_state(17) = typecast(Buffer(73:76),'single');
                        lastsys_state(18) = typecast(Buffer(77:80),'single');
                        lastsys_state(19) = typecast(Buffer(81:84),'single');
                        lastsys_state(20) = typecast(Buffer(85:88),'single');
                        lastsys_state(21) = typecast(Buffer(89:92),'single');
                        lastsys_state(22) = typecast(Buffer(93:96),'single');
                        lastsys_state(23) = typecast(Buffer(97:100),'single');
                    case 81
                        %% 解析MSG_UNIX_TIME
                        lastunix_time(1) = typecast(Buffer(1:4),'uint32');
                        lastunix_time(2) = typecast(Buffer(5:8),'uint32');
                    case 82
                        %% 解析MSG_FORMAT_TIME
                        lastformat_time(1) = typecast(Buffer(1:4),'uint32');
                        lastformat_time(2) = typecast(Buffer(5:6),'uint16');
                        lastformat_time(3) = typecast(Buffer(7:8),'uint16');
                        lastformat_time(4) = typecast(Buffer(9:9),'uint8');
                        lastformat_time(5) = typecast(Buffer(10:10),'uint8');
                        lastformat_time(6) = typecast(Buffer(11:11),'uint8');
                        lastformat_time(7) = typecast(Buffer(12:12),'uint8');
                        lastformat_time(8) = typecast(Buffer(13:13),'uint8');
                        lastformat_time(9) = typecast(Buffer(14:14),'uint8');
                    case 83
                        %% 解析MSG_STATUS
                        laststatus(1) = typecast(Buffer(1:2),'uint16');
                        laststatus(2) = typecast(Buffer(3:4),'uint16');
                    case 84
                        %% 解析MSG_POS_STD_DEV
                        lastpos_std_dev(1) =  typecast(Buffer(1:4),'single');
                        lastpos_std_dev(2) =  typecast(Buffer(5:8),'single');
                        lastpos_std_dev(3) =  typecast(Buffer(9:12),'single');
                    case 85
                        %% 解析MSG_VEL_STD_DEV
                        lastvel_std_dev(1) =  typecast(Buffer(1:4),'single');
                        lastvel_std_dev(2) =  typecast(Buffer(5:8),'single');
                        lastvel_std_dev(3) =  typecast(Buffer(9:12),'single');
                    case 86
                        %% 解析MSG_EULER_ORIEN_STD_DEV
                        lasteuler_orien_std_dev(1) =  typecast(Buffer(1:4),'single');
                        lasteuler_orien_std_dev(2) =  typecast(Buffer(5:8),'single');
                        lasteuler_orien_std_dev(3) =  typecast(Buffer(9:12),'single');
                    case 87
                        %% 解析MSG_QUAT_ORIEN_STD_DEV
                        lastquat_orien_std_dev(1) =  typecast(Buffer(1:4),'single');
                        lastquat_orien_std_dev(2) =  typecast(Buffer(5:8),'single');
                        lastquat_orien_std_dev(3) =  typecast(Buffer(9:12),'single');
                        lastquat_orien_std_dev(4) =  typecast(Buffer(13:16),'single');
                    case 88
                        %% 解析MSG_RAW_SENSORS
                        lastraw_sensors(1) = typecast(Buffer(1:4),'single');
                        lastraw_sensors(2) = typecast(Buffer(5:8),'single');
                        lastraw_sensors(3) = typecast(Buffer(9:12),'single');
                        lastraw_sensors(4) = typecast(Buffer(13:16),'single');
                        lastraw_sensors(5) = typecast(Buffer(17:20),'single');
                        lastraw_sensors(6) = typecast(Buffer(21:24),'single');
                        lastraw_sensors(7) = typecast(Buffer(25:28),'single');
                        lastraw_sensors(8) = typecast(Buffer(29:32),'single');
                        lastraw_sensors(9) = typecast(Buffer(33:36),'single');
                        lastraw_sensors(10) = typecast(Buffer(37:40),'single');
                        lastraw_sensors(11) = typecast(Buffer(41:44),'single');
                        lastraw_sensors(12) = typecast(Buffer(45:48),'single');
                    case 89
                        %% 解析MSG_RAW_GNSS
                        lastraw_gnss(1) = typecast(Buffer(1:4),'uint32');
                        lastraw_gnss(2) = typecast(Buffer(5:8),'uint32');
                        lastraw_gnss(3) = typecast(Buffer(9:16),'double');
                        lastraw_gnss(4) = typecast(Buffer(17:24),'double');
                        lastraw_gnss(5) = typecast(Buffer(25:32),'double');
                        lastraw_gnss(6) = typecast(Buffer(33:36),'single');
                        lastraw_gnss(7) = typecast(Buffer(37:40),'single');
                        lastraw_gnss(8) = typecast(Buffer(41:44),'single');
                        lastraw_gnss(9) = typecast(Buffer(45:48),'single');
                        lastraw_gnss(10) = typecast(Buffer(49:52),'single');
                        lastraw_gnss(11) = typecast(Buffer(53:56),'single');
                    case 90
                        %% 解析MSG_SATELLITE
                        lastsatellite(1) = typecast(Buffer(1:4),'single');
                        lastsatellite(2) = typecast(Buffer(5:8),'single');
                        lastsatellite(3) = typecast(Buffer(9:9),'uint8');
                    case 92
                        %% 解析MSG_GEODETIC_POS
                        lastgeodetic_pos(1) = typecast(Buffer(1:8),'double');
                        lastgeodetic_pos(2) = typecast(Buffer(9:16),'double');
                        lastgeodetic_pos(3) = typecast(Buffer(17:24),'double');
                        lastgeodetic_pos(4) = typecast(Buffer(25:28),'single');
                        lastgeodetic_pos(5) = typecast(Buffer(29:32),'single');
                    case 93
                        %% 解析MSG_ECEF_POS
                        lastecef_pos(1) = typecast(Buffer(1:8),'double');
                        lastecef_pos(2) = typecast(Buffer(9:16),'double');
                        lastecef_pos(3) = typecast(Buffer(17:24),'double');
                    case 94
                        %% 解析MSG_UTM_POS
                        lastutm_pos(1) = typecast(Buffer(1:4),'single');
                        lastutm_pos(2) = typecast(Buffer(5:8),'single');
                        lastutm_pos(3) = typecast(Buffer(9:12),'single');
                        lastutm_pos(4) = typecast(Buffer(13:13),'uint8');
                        lastutm_pos(5) = typecast(Buffer(14:14),'int8');
                    case 95
                        %% 解析MSG_NED_VEL
                        lastned_vel(1) = typecast(Buffer(1:4),'single');
                        lastned_vel(2) = typecast(Buffer(5:8),'single');
                        lastned_vel(3) = typecast(Buffer(9:12),'single');
                    case 96
                        %% 解析MSG_BODY_VEL
                        lastbody_vel(1) = typecast(Buffer(1:4),'single');
                        lastbody_vel(2) = typecast(Buffer(5:8),'single');
                        lastbody_vel(3) = typecast(Buffer(9:12),'single');
                    case 97
                        %% 解析MSG_ACCELERATION
                        lastacceleration(1) = typecast(Buffer(1:4),'single');
                        lastacceleration(2) = typecast(Buffer(5:8),'single');
                        lastacceleration(3) = typecast(Buffer(9:12),'single');
                    case 98
                        %% 解析MSG_BODY_ACCELERATION
                        lastbody_acceleration(1) = typecast(Buffer(1:4),'single');
                        lastbody_acceleration(2) = typecast(Buffer(5:8),'single');
                        lastbody_acceleration(3) = typecast(Buffer(9:12),'single');
                        lastbody_acceleration(4) = typecast(Buffer(13:16),'single');
                    case 99
                        %% 解析MSG_EULER_ORIEN
                        lasteuler_orien(1) = typecast(Buffer(1:4),'single');
                        lasteuler_orien(2) = typecast(Buffer(5:8),'single');
                        lasteuler_orien(3) = typecast(Buffer(9:12),'single');
                    case 100
                        %% 解析MSG_QUAT_ORIEN
                        lastquat_orien(1) = typecast(Buffer(1:4),'single');
                        lastquat_orien(2) = typecast(Buffer(5:8),'single');
                        lastquat_orien(3) = typecast(Buffer(9:12),'single');
                        lastquat_orien(4) = typecast(Buffer(13:16),'single');
                    case 101
                        %% 解析MSG_DCM_ORIEN
                        lastdcm_orien(1) = typecast(Buffer(1:4),'single');
                        lastdcm_orien(2) = typecast(Buffer(5:8),'single');
                        lastdcm_orien(3) = typecast(Buffer(9:12),'single');
                        lastdcm_orien(4) = typecast(Buffer(13:16),'single');
                        lastdcm_orien(5) = typecast(Buffer(17:20),'single');
                        lastdcm_orien(6) = typecast(Buffer(21:24),'single');
                        lastdcm_orien(7) = typecast(Buffer(25:28),'single');
                        lastdcm_orien(8) = typecast(Buffer(29:32),'single');
                        lastdcm_orien(9) = typecast(Buffer(33:36),'single');
                    case 102
                        %% 解析MSG_ANGULAR_VEL
                        lastangular_vel(1) = typecast(Buffer(1:4),'single');
                        lastangular_vel(2) = typecast(Buffer(5:8),'single');
                        lastangular_vel(3) = typecast(Buffer(9:12),'single');
                    case 103
                        %% 解析MSG_ANGULAR_ACC
                        lastangular_acc(1) = typecast(Buffer(1:4),'single');
                        lastangular_acc(2) = typecast(Buffer(5:8),'single');
                        lastangular_acc(3) = typecast(Buffer(9:12),'single');
                    case 109
                        %% 解析MSG_RUNNING_TIME
                        lastrunning_time(1) = typecast(Buffer(1:4),'uint32');
                        lastrunning_time(2) = typecast(Buffer(5:8),'uint32');
                    case 110
                        %% 解析MSG_LOCAL_MAG_FIELD
                        lastlocal_mag_field(1) = typecast(Buffer(1:4),'single');
                        lastlocal_mag_field(2) = typecast(Buffer(5:8),'single');
                        lastlocal_mag_field(3) = typecast(Buffer(9:12),'single');
                        lastlocal_mag_field(4) = typecast(Buffer(13:16),'single');
                        lastlocal_mag_field(5) = typecast(Buffer(17:20),'single');
                        lastlocal_mag_field(6) = typecast(Buffer(21:24),'single');
                    case 111
                        %% 解析MSG_ODOMETER_STATE
                        lastodometer_state(1) = typecast(Buffer(1:4),'int32');
                        lastodometer_state(2) = typecast(Buffer(5:8),'single');
                        lastodometer_state(3) = typecast(Buffer(9:12),'single');
                        lastodometer_state(4) = typecast(Buffer(13:16),'single');
                        lastodometer_state(5) = typecast(Buffer(17:17),'uint8');
                        lastodometer_state(6) = typecast(Buffer(18:18),'uint8');
                    case 114
                        %% 解析MSG_GEOID_HEIGHT
                        lastgeoid_height(1) = typecast(Buffer(1:4),'single');
                    case 117
                        %% 解析MSG_WIND
                        lastwind(1) = typecast(Buffer(1:4),'single');
                        lastwind(2) = typecast(Buffer(5:8),'single');
                        lastwind(3) = typecast(Buffer(9:12),'single');
                    case 118
                        %% 解析MSG_HEAVE
                        lastheave(1) = typecast(Buffer(1:4),'single');
                        lastheave(2) = typecast(Buffer(5:8),'single');
                        lastheave(3) = typecast(Buffer(9:12),'single');
                        lastheave(4) = typecast(Buffer(13:16),'single');
                    case 120
                        %% 解析MSG_GNSS_DUAL_ANT
                        lastgnss_dual_ant(1) = typecast(Buffer(1:4),'uint32');
                        lastgnss_dual_ant(2) = typecast(Buffer(5:12),'double');
                        lastgnss_dual_ant(3) = typecast(Buffer(13:20),'double');
                        lastgnss_dual_ant(4) = typecast(Buffer(21:28),'double');
                        lastgnss_dual_ant(5) = typecast(Buffer(29:36),'double');
                        lastgnss_dual_ant(6) = typecast(Buffer(37:44),'double');
                        lastgnss_dual_ant(7) = typecast(Buffer(45:52),'double');
                        lastgnss_dual_ant(8) = typecast(Buffer(53:60),'double');
                        lastgnss_dual_ant(9) = typecast(Buffer(61:68),'double');
                        lastgnss_dual_ant(10) = typecast(Buffer(69:72),'single');
                        lastgnss_dual_ant(11) = typecast(Buffer(73:76),'single');
                        lastgnss_dual_ant(12) = typecast(Buffer(77:80),'single');
                        lastgnss_dual_ant(13) = typecast(Buffer(81:88),'double');
                        lastgnss_dual_ant(14) = typecast(Buffer(89:96),'double');
                        lastgnss_dual_ant(15) = typecast(Buffer(97:100),'single');
                        lastgnss_dual_ant(16) = typecast(Buffer(101:104),'single');
                        lastgnss_dual_ant(17) = typecast(Buffer(105:108),'single');
                        lastgnss_dual_ant(18) = typecast(Buffer(109:116),'double');
                        lastgnss_dual_ant(19) = typecast(Buffer(117:120),'single');
                        lastgnss_dual_ant(20) = typecast(Buffer(121:128),'double');
                        lastgnss_dual_ant(21) = typecast(Buffer(129:132),'single');
                        lastgnss_dual_ant(22) = typecast(Buffer(133:133),'uint8');
                        lastgnss_dual_ant(23) = typecast(Buffer(134:134),'uint8');
                    case 122
                        %% 解析MSG_GIMBAL_STATE
                        lastgimbal_state(1) = typecast(Buffer(1:4),'single');
                        lastgimbal_state(2) = typecast(Buffer(5:8),'uint32');
                    case 123
                        %% 解析MSG_AUTOMOTIVE
                        lastautomotive(1) = typecast(Buffer(1:4),'single');
                        lastautomotive(2) = typecast(Buffer(5:8),'single');
                        lastautomotive(3) = typecast(Buffer(9:12),'single');
                        lastautomotive(4) = typecast(Buffer(13:16),'single');
                        lastautomotive(5) = typecast(Buffer(17:20),'single');
                        lastautomotive(6) = typecast(Buffer(21:24),'uint32');
                    case 128
                        %% 解析MSG_INSTALL_ALIGN
                        lastinstall_align(1) = typecast(Buffer(1:1),'uint8');
                        lastinstall_align(2) = typecast(Buffer(2:5),'single');
                        lastinstall_align(3) = typecast(Buffer(6:9),'single');
                        lastinstall_align(4) = typecast(Buffer(10:13),'single');
                        lastinstall_align(5) = typecast(Buffer(14:17),'single');
                        lastinstall_align(6) = typecast(Buffer(18:21),'single');
                        lastinstall_align(7) = typecast(Buffer(22:25),'single');
                        lastinstall_align(8) = typecast(Buffer(26:29),'single');
                        lastinstall_align(9) = typecast(Buffer(30:33),'single');
                        lastinstall_align(10) = typecast(Buffer(34:37),'single');
                        lastinstall_align(11) = typecast(Buffer(38:41),'single');
                    case 129
                        %% 解析MSG_FILTER_OPTIONS
                        lastfilter_options(1) = typecast(Buffer(1:1),'uint8');
                        lastfilter_options(2) = typecast(Buffer(2:2),'uint8');
                        lastfilter_options(3) = typecast(Buffer(3:3),'uint8');
                        lastfilter_options(4) = typecast(Buffer(4:4),'uint8');
                        lastfilter_options(5) = typecast(Buffer(5:5),'uint8');
                        lastfilter_options(6) = typecast(Buffer(6:6),'uint8');
                        lastfilter_options(7) = typecast(Buffer(7:7),'uint8');
                        lastfilter_options(8) = typecast(Buffer(8:8),'uint8');
                        lastfilter_options(9) = typecast(Buffer(9:9),'uint8');
                        lastfilter_options(10) = typecast(Buffer(10:10),'uint8');
                        lastfilter_options(11) = typecast(Buffer(11:11),'uint8');
                        lastfilter_options(12) = typecast(Buffer(12:12),'uint8');
                        lastfilter_options(13) = typecast(Buffer(13:13),'uint8');
                        lastfilter_options(14) = typecast(Buffer(10:10),'uint8');
                        lastfilter_options(15) = typecast(Buffer(11:11),'uint8');
                        lastfilter_options(16) = typecast(Buffer(12:12),'uint8');
                        lastfilter_options(17) = typecast(Buffer(13:13),'uint8');
                        lastfilter_options(18) = typecast(Buffer(14:14),'uint8');
                        lastfilter_options(19) = typecast(Buffer(15:15),'uint8');
                        lastfilter_options(20) = typecast(Buffer(16:16),'uint8');
                        lastfilter_options(21) = typecast(Buffer(17:17),'uint8');
                end
            end
            FStatus = 0;
    end
end

imu = lastimu;
ahrs = lastahrs;
ins_gps = lastins_Gps;
sys_state =   lastsys_state;
unix_time =    lastunix_time;
format_time = lastformat_time;
status =  laststatus;
pos_std_dev=lastpos_std_dev;
vel_std_dev=lastvel_std_dev;
euler_orien_std_dev= lasteuler_orien_std_dev;
quat_orien_std_dev=lastquat_orien_std_dev;
raw_sensors=lastraw_sensors;
raw_gnss=lastraw_gnss;
satellite=lastsatellite;
geodetic_pos=lastgeodetic_pos;
ecef_pos=lastecef_pos;
utm_pos=lastutm_pos;
ned_vel=lastned_vel;
body_vel= lastbody_vel;
acceleration=lastacceleration;
body_acceleration=lastbody_acceleration;
euler_orien=lasteuler_orien;
quat_orien=lastquat_orien;
dcm_orien=lastdcm_orien;
angular_vel=lastangular_vel;
angular_acc=lastangular_acc;
running_time= lastrunning_time;
local_mag_field= lastlocal_mag_field;
odometer_state= lastodometer_state;
geoid_height=lastgeoid_height;
wind=lastwind ;
heave=lastheave;
gnss_dual_ant=lastgnss_dual_ant;
gimbal_state=lastgimbal_state;
automotive= lastautomotive;
install_align=lastinstall_align;
filter_options= lastfilter_options;

end
